simulink model "irobotcomunication"  (Simulink 7.0)
settings: Solver=FixedStepDiscrete  StartTime=0.0  StopTime=100  FixedStep=0.1  RelTol=1e-3
libraries: vrlib x1, utility x1
settings Model: Creator=tdlehman  LastModifiedBy=root  ExtModeAutoUpdateStatusClock=off
settings OptimizationCC: LocalBlockOutputs=off
settings DebuggingCC: AlgebraicLoopMsg=none  MultiTaskCondExecSysMsg=warning
settings RTWCC: SystemTargetFile=rtai.tlc  GenCodeOnly=on  TemplateMakefile=rtai.tmf  Description=Linux RTAI Real-Time Target  ProcessScript=rtai_make_rtw_hook  CustomInclude=./lqry/lqry
settings RTWCC: CustomSource=|
  | balgbk.o d1nrm.o dgefam.o drot.o dswap.o gradbk.o lineq.o mlineq.o mqfwo.o mulb.o
  | orthes.o qzval.o rinv.o scalbk.o symslv.o balgen.o daxpy.o dgeslm.o dscal.o exchqz.o
  | gradeq.o lypcnd.o mmul.o mscale.o mulwoa.o ortran.o reduce.o rotc.o scaleg.o trnata.o
  | cmprs.o ddot.o dnrm2.o dstslv.o fbgain.o hqrort.o lypdsd.o mqfa.o msub.o newt.o qzhesw.o
  | resid.o rotr.o sepest.o trnatb.o creg.o dgecom.o drotg.o dsvdc.o giv.o madd.o mqf.o
  | mula.o order.o qzitw.o ricsol.o save.o symprd.o xty.o
settings STFCustomTargetCC: GenFloatMathFcnCalls=ANSI_C  ModelReferenceCompliant=off  MatFileLogging=on  SystemTargetFile=rtai.tlc

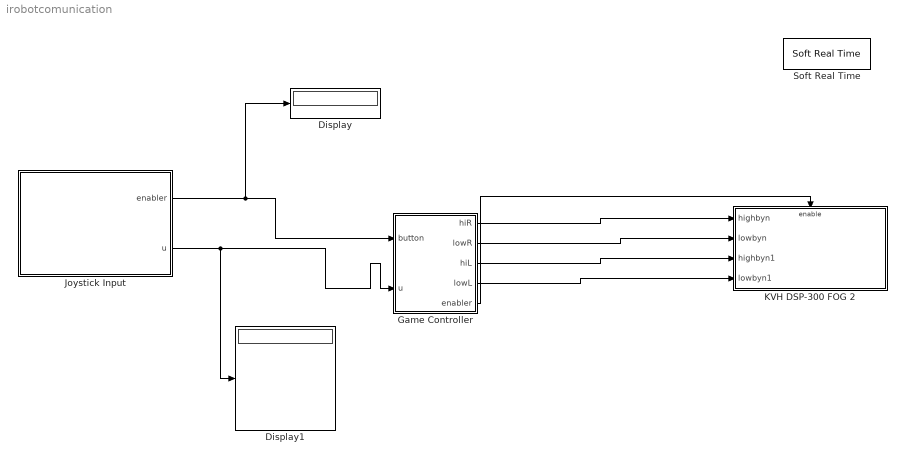
== system irobotcomunication ==
  Display : Display
  Display1 : Display
  Game Controller : Stateflow chart
  Joystick Input : Subsystem
  KVH DSP-300 FOG 2 : Subsystem  mask(EZServo){port=COM1, baudrate=57600, databit=8, stopbit=1, parity=None, samptime=0.1}
      mask prompts: baudrate "Baud rate:"; databit "Number of data bits:"; stopbit "Number of stop bits:"; samptime "Sample Time:"
      mask help:
      | iRobot Create
      | (Alessio Grompone)
      |
      | Select the following options for standard use:
      |
      | 57600 bps, 8 Data Bits, 1 Stop Bit, No Parity, No Protocol
      mask StyleString: popup(COM1|COM2|COM3|COM4|COM5|COM6|COM7|COM8),popup(115200|57600|38400|19200|9600|4800|2400|1200|300|110),popup(8|7|6|5),popup(1|2),popup(None|Odd|Even),edit
      mask Display:
      | disp('iRobot \n Create');
      | 
      | 
      | 
      | port_label('input',1,'Command 1')
      | port_label('input',2,'Command 2')
      | port_label('input',3,'Command 3')
      | port_label('input',4,'Command 4')
  Soft Real Time : utility/Soft Real Time  x=1
  wires:
  Game Controller/1(hiR) -> KVH DSP-300 FOG 2/1(highbyn)
  Game Controller/2(lowR) -> KVH DSP-300 FOG 2/2(lowbyn)
  Game Controller/3(hiL) -> KVH DSP-300 FOG 2/3(highbyn1)
  Game Controller/4(lowL) -> KVH DSP-300 FOG 2/4(lowbyn1)
  Game Controller/5(enabler) -> KVH DSP-300 FOG 2/Enable
  Joystick Input/2(u) -> Game Controller/2(u), Display1/1
  Joystick Input/1(enabler) -> Game Controller/1(button), Display/1

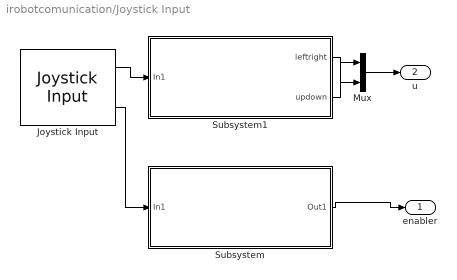
== system irobotcomunication/Joystick Input ==
  Joystick Input : vrlib/Joystick Input  joyid=1  adjustports=on  forcefeed=off
  Mux : Mux  Inputs=2
  Subsystem : Subsystem
  Subsystem1 : Subsystem
  enabler : Outport  OutDataType=sfix(16)  OutScaling=2^0
  u : Outport  Port=2  OutDataType=sfix(16)  OutScaling=2^0
  wires:
  Joystick Input/1 -> Subsystem1/1(In1)
  Joystick Input/2 -> Subsystem/1(In1)
  Subsystem/1(Out1) -> enabler/1
  Mux/1 -> u/1
  Subsystem1/1(leftright) -> Mux/2
  Subsystem1/2(updown) -> Mux/1

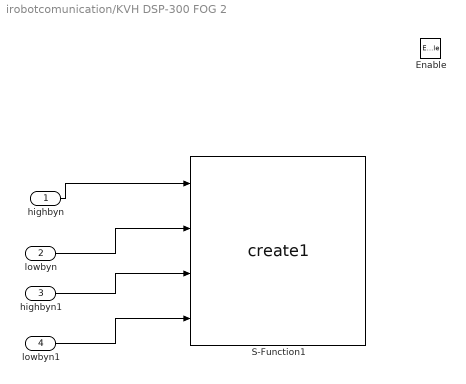
== system irobotcomunication/KVH DSP-300 FOG 2 ==
  highbyn : Inport  OutDataType=sfix(16)  OutScaling=2^0
  lowbyn : Inport  Port=2  OutDataType=sfix(16)  OutScaling=2^0
  highbyn1 : Inport  Port=3  OutDataType=sfix(16)  OutScaling=2^0
  lowbyn1 : Inport  Port=4  OutDataType=sfix(16)  OutScaling=2^0
  Enable : EnablePort
  S-Function1 : S-Function  FunctionName=create1  Parameters=port, baudrate, databit, stopbit, parity, samptime
  wires:
  highbyn/1 -> S-Function1/1
  lowbyn/1 -> S-Function1/2
  highbyn1/1 -> S-Function1/3
  lowbyn1/1 -> S-Function1/4

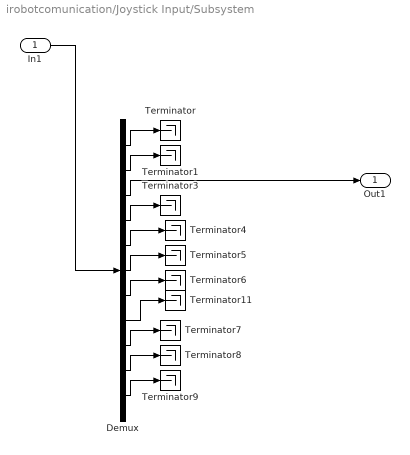
== system irobotcomunication/Joystick Input/Subsystem ==
  In1 : Inport  OutDataType=sfix(16)  OutScaling=2^0
  Demux : Demux  Outputs=11
  Terminator{,1,3..9,11} (10 alike) : Terminator
  Out1 : Outport  OutDataType=sfix(16)  OutScaling=2^0
  wires:
  In1/1 -> Demux/1
  Demux/1 -> Terminator/1
  Demux/2 -> Terminator1/1
  Demux/3 -> Out1/1
  Demux/4 -> Terminator3/1
  Demux/5 -> Terminator4/1
  Demux/9 -> Terminator7/1
  Demux/10 -> Terminator8/1
  Demux/11 -> Terminator9/1
  Demux/6 -> Terminator5/1
  Demux/7 -> Terminator6/1
  Demux/8 -> Terminator11/1

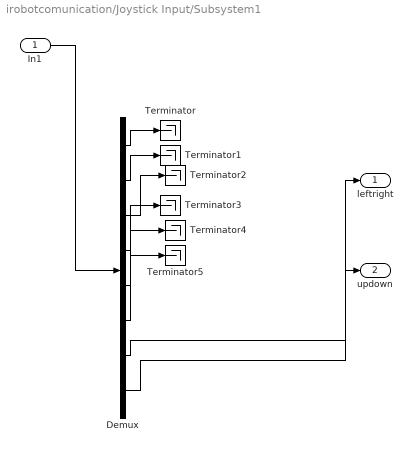
== system irobotcomunication/Joystick Input/Subsystem1 ==
  In1 : Inport  OutDataType=sfix(16)  OutScaling=2^0
  Demux : Demux  Outputs=8
  Terminator{,1..5} (6 alike) : Terminator
  leftright : Outport  OutDataType=sfix(16)  OutScaling=2^0
  updown : Outport  Port=2  OutDataType=sfix(16)  OutScaling=2^0
  wires:
  Demux/8 -> updown/1
  Demux/7 -> leftright/1
  Demux/6 -> Terminator5/1
  Demux/5 -> Terminator4/1
  Demux/4 -> Terminator3/1
  Demux/2 -> Terminator1/1
  Demux/1 -> Terminator/1
  In1/1 -> Demux/1
  Demux/3 -> Terminator2/1

== matlab function Game Controller ==
  data: button input inherited; u input inherited; hiR output inherited; lowR output inherited; hiL output inherited; lowL output inherited; enabler output inherited
function [hiR,lowR,hiL,lowL,enabler] = fcn(button,u)
% This block supports the Embedded MATLAB subset.
% See the help menu for details. 


if u(2)==1; %turn right

hiR=0;
lowR=0;
hiL=12;
lowL=8;

elseif u(2)==-1;%turn left
    
hiR=12;
lowR=8;
hiL=0;
lowL=0;

else
    
if u(1)==1; %backwards

hiR=255;
lowR=56;
hiL=255;
lowL=56;

elseif u(1)==-1;%forward
    
hiR=12;
lowR=8;
hiL=12;
lowL=8;

else %stop
    
hiR=0;
lowR=0;
hiL=0;
lowL=0;  

end 

end

if button==1;
    
    enabler=1;
    
else
    enabler=0;
end
